simulink model "BitwiseOperator"  (R2018b)
settings: Solver=FixedStepDiscrete  StartTime=0.0  StopTime=10.0  RelTol=1e-3
libraries: simulink x5
settings Model: Creator=lenovo2  LastModifiedBy=lenovo2
settings OptimizationCC: DefaultParameterBehavior=Inlined  EnhancedBackFolding=on  PassReuseOutputArgsAs=Individual arguments  OptimizeBlockOrder=speed  DifferentSizesBufferReuse=on  OptimizationCustomize=off
settings DebuggingCC: UnderspecifiedInitializationDetection=Classic  MergeDetectMultiDrivingBlocksExec=none  ParameterTunabilityLossMsg=error
settings ModelReferenceCC: PropagateSignalLabelsOutOfModel=off
settings SFSimCC: MATLABDynamicMemAlloc=off
settings RTWCC: SystemTargetFile=ert.tlc  GenCodeOnly=on  TemplateMakefile=ert_default_tmf  GenerateReport=on  IncludeHyperlinkInReport=on  LaunchReport=on  GenerateTraceInfo=on  GenerateTraceReport=on  GenerateTraceReportSl=on  GenerateTraceReportSf=on  GenerateTraceReportEml=on
settings CodeAppCC: ForceParamTrailComments=on  IgnoreCustomStorageClasses=off  OperatorAnnotations=on  SimulinkDataObjDesc=on  SFDataObjDesc=on  InsertBlockDesc=on
settings ERTTargetCC: TargetLangStandard=C99 (ISO)  GenerateSampleERTMain=on  InlinedParameterPlacement=NonHierarchical  ERTCustomFileTemplate=example_file_process.tlc

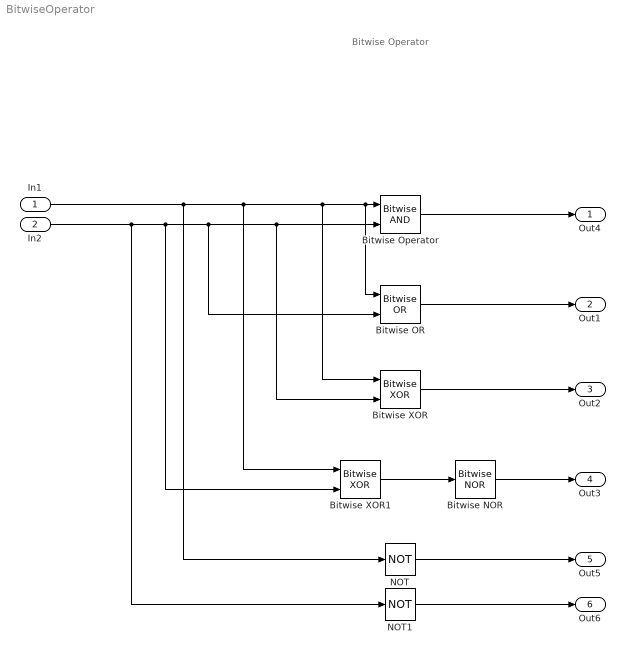
== system BitwiseOperator ==
  note: Bitwise Operator
  In1 : Inport
  In2 : Inport  Port=2
  Bitwise Operator : simulink/Logic and Bit Operations/Bitwise Operator  logicop=AND  UseBitMask=off  NumInputPorts=2  BitMask=bin2dec('11011000')  BitMaskRealWorld=Stored Integer
  Bitwise NOR : simulink/Logic and Bit Operations/Bitwise Operator  logicop=NOR  UseBitMask=off  BitMask=bin2dec('11011001')  BitMaskRealWorld=Stored Integer
  Bitwise OR : simulink/Logic and Bit Operations/Bitwise Operator  logicop=OR  UseBitMask=off  NumInputPorts=2  BitMask=bin2dec('11011001')  BitMaskRealWorld=Stored Integer
  Bitwise XOR : simulink/Logic and Bit Operations/Bitwise Operator  logicop=XOR  UseBitMask=off  NumInputPorts=2  BitMask=bin2dec('11011001')  BitMaskRealWorld=Stored Integer
  Bitwise XOR1 : simulink/Logic and Bit Operations/Bitwise Operator  logicop=XOR  UseBitMask=off  NumInputPorts=2  BitMask=bin2dec('11011001')  BitMaskRealWorld=Stored Integer
  NOT : Logic  Operator=NOT  IconShape=distinctive  AllPortsSameDT=off  OutDataTypeStr=boolean
  NOT1 : Logic  Operator=NOT  IconShape=distinctive  AllPortsSameDT=off  OutDataTypeStr=boolean
  Out4 : Outport  OutDataTypeStr=boolean
  Out1 : Outport  Port=2  OutDataTypeStr=boolean
  Out2 : Outport  Port=3  OutDataTypeStr=boolean
  Out3 : Outport  Port=4  OutDataTypeStr=boolean
  Out5 : Outport  Port=5  OutDataTypeStr=boolean
  Out6 : Outport  Port=6  OutDataTypeStr=boolean
  wires:
  In1/1 -> NOT/1, Bitwise XOR1/1, Bitwise XOR/1, Bitwise OR/1, Bitwise Operator/1
  Bitwise Operator/1 -> Out4/1
  In2/1 -> NOT1/1, Bitwise XOR1/2, Bitwise OR/2, Bitwise XOR/2, Bitwise Operator/2
  Bitwise OR/1 -> Out1/1
  Bitwise XOR/1 -> Out2/1
  Bitwise XOR1/1 -> Bitwise NOR/1
  Bitwise NOR/1 -> Out3/1
  NOT/1 -> Out5/1
  NOT1/1 -> Out6/1
